simulink model "pendule_inv_echant_etu"  (R2022a)
settings: Solver=VariableStepAuto  StartTime=0.0  StopTime=10.0  RelTol=1e-3
values from neighbouring files (symbols this model uses):
  g = 9.81    [simu_pendule_inv_capteur_etu.m]
  K = [10 1]    [simu_pendule_inv_capteur_etu.m]
  l = 10    [simu_pendule_inv_capteur_etu.m]
  ue = 0    [simu_pendule_inv_capteur_etu.m]
  xe = [0 0]'    [simu_pendule_inv_capteur_etu.m]
undefined symbols (not defined in the file or in its folder): delta_t, DiscIntNeverNeededParam, x0
settings Model: Creator=melallem  LastModifiedBy=elgue
settings DebuggingCC: UnconnectedInputMsg=warning  UnconnectedOutputMsg=warning  UnconnectedLineMsg=warning
settings RTWCC: DLArmComputeVersion=19.05

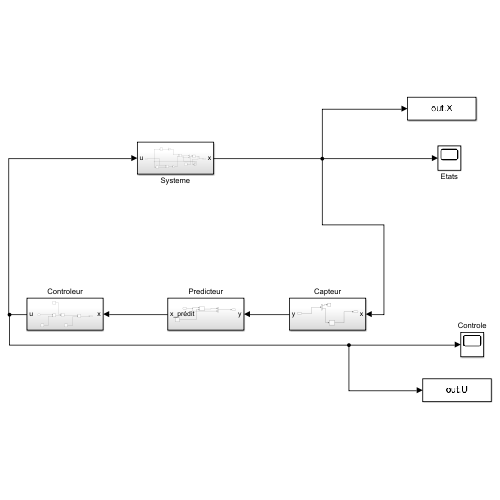
[thumbnail: Simulink's stored preview of the top-level diagram]
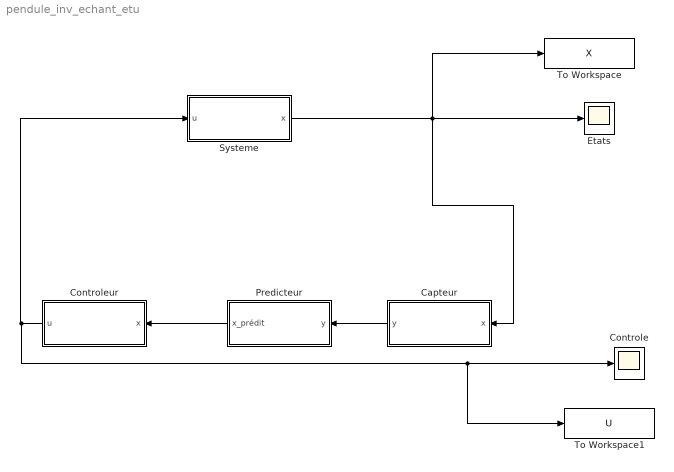
== system pendule_inv_echant_etu ==
  Capteur : Subsystem
  Controle : Scope
  Controleur : Subsystem
  Etats : Scope
  Predicteur : Subsystem
  Systeme : Subsystem
  To Workspace : ToWorkspace  VariableName=X  SaveFormat=Timeseries  SampleTime=-1
  To Workspace1 : ToWorkspace  VariableName=U  SaveFormat=Timeseries  SampleTime=-1
  wires:
  Capteur/1(y) -> Predicteur/1(y)
  Predicteur/1(x_prédit) -> Controleur/1(x)
  Systeme/1(x) -> Capteur/1(x), Etats/1, To Workspace/1
  Controleur/1(u) -> To Workspace1/1, Controle/1, Systeme/1(u)

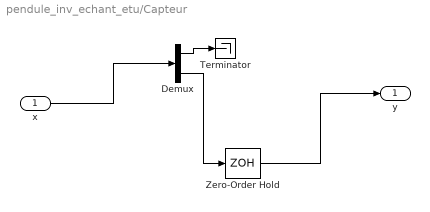
== system pendule_inv_echant_etu/Capteur ==
  x : Inport
  Demux : Demux  Outputs=2
  Terminator : Terminator
  Zero-Order Hold : ZeroOrderHold  SampleTime=delta_t
  y : Outport
  wires:
  x/1 -> Demux/1
  Demux/1 -> Terminator/1
  Demux/2 -> Zero-Order Hold/1
  Zero-Order Hold/1 -> y/1

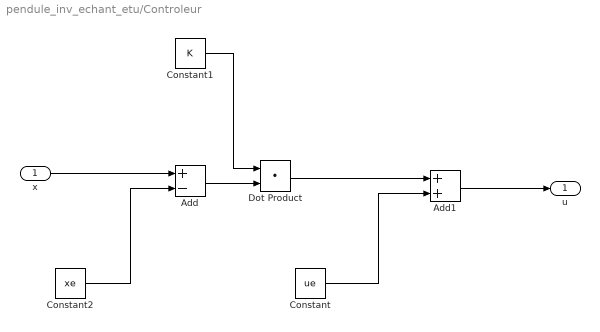
== system pendule_inv_echant_etu/Controleur ==
  x : Inport
  Add : Sum  Inputs=+-
  Add1 : Sum
  Constant : Constant  Value=ue
  Constant1 : Constant  Value=K
  Constant2 : Constant  Value=xe
  Dot Product : DotProduct  OutDataTypeStr=Inherit: Inherit via internal rule
  u : Outport
  wires:
  x/1 -> Add/1
  Constant2/1 -> Add/2
  Add/1 -> Dot Product/2
  Constant1/1 -> Dot Product/1
  Dot Product/1 -> Add1/1
  Constant/1 -> Add1/2
  Add1/1 -> u/1

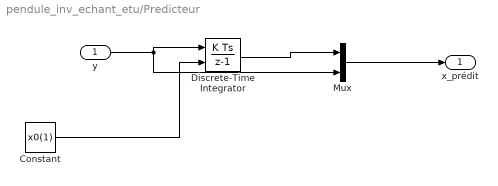
== system pendule_inv_echant_etu/Predicteur ==
  y : Inport
  Constant : Constant  Value=x0(1)
  Discrete-Time Integrator : DiscreteIntegrator  InitialConditionSource=external  SampleTime=-1  ICPrevOutput=DiscIntNeverNeededParam  ICPrevScaledInput=DiscIntNeverNeededParam
  Mux : Mux  Inputs=2
  x_prédit : Outport
  wires:
  y/1 -> Mux/2, Discrete-Time Integrator/1
  Discrete-Time Integrator/1 -> Mux/1
  Mux/1 -> x_prédit/1
  Constant/1 -> Discrete-Time Integrator/2

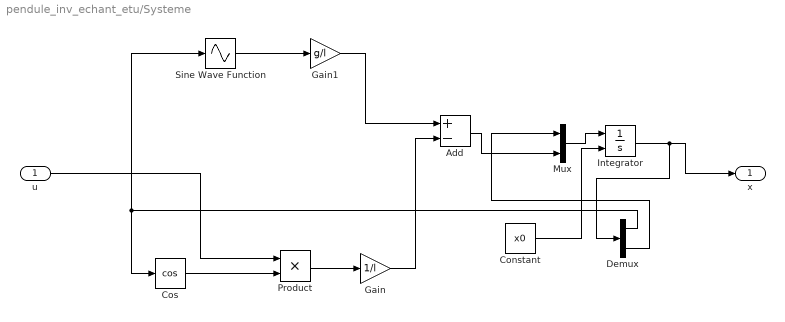
== system pendule_inv_echant_etu/Systeme ==
  u : Inport
  Add : Sum  Inputs=+-
  Constant : Constant  Value=x0
  Cos : Trigonometry  Operator=cos
  Demux : Demux  Outputs=2
  Gain : Gain  Gain=1/l
  Gain1 : Gain  Gain=g/l
  Integrator : Integrator  InitialConditionSource=external
  Mux : Mux  Inputs=2
  Product : Product
  Sine Wave Function : Sin  TimeSource=Use external signal  SampleTime=0
  x : Outport
  wires:
  u/1 -> Product/1
  Demux/2 -> Mux/1
  Product/1 -> Gain/1
  Cos/1 -> Product/2
  Demux/1 -> Cos/1, Sine Wave Function/1
  Sine Wave Function/1 -> Gain1/1
  Gain1/1 -> Add/1
  Gain/1 -> Add/2
  Add/1 -> Mux/2
  Mux/1 -> Integrator/1
  Integrator/1 -> Demux/1, x/1
  Constant/1 -> Integrator/2
